simulink model "Arduino_observador_2021"  (R2021a)
settings: Solver=ode4  StartTime=0.0  StopTime=inf  FixedStep=0.001  RelTol=1e-3  EnableMultiTasking=on
values from neighbouring files (symbols this model uses):
  A = [-Ra/La -Kg/(Kt*La) ... (first row only)    [observador_arduino.m]
  B = [1/La ; 0]    [observador_arduino.m]
  C = [0 1]    [observador_arduino.m]
  K = [K1 K2]    [observador_arduino.m]
  ki = double(solve(coeffs_det_A_r(end-3)==pol_caract(4), ki))    [observador_arduino.m]
  L = place(A', C', desired_poles)'    [observador_arduino.m]
libraries: arduinolib x2
settings Model: SILPILModeSetting=veronly  ExtModeTrigDuration=2  Creator=lcauf  LastModifiedBy=carol
settings OptimizationCC: EnhancedBackFolding=on  PassReuseOutputArgsAs=Individual arguments  ZeroExternalMemoryAtStartup=off  ZeroInternalMemoryAtStartup=off  MaxStackSize=64  OptimizeBlockOrder=speed  DifferentSizesBufferReuse=on  OptimizationCustomize=off  EfficientTunableParamExpr=on
settings DebuggingCC: ParameterTunabilityLossMsg=error
settings HardwareCC: ProdBitPerPointer=32  ProdBitPerSizeT=32  ProdBitPerPtrDiffT=32  ProdLargestAtomicInteger=Long  ProdLargestAtomicFloat=Double  ProdWordSize=32  ProdHWDeviceType=ARM Compatible->ARM Cortex  UseEmbeddedCoderFeatures=off
settings SFSimCC: MATLABDynamicMemAlloc=off
settings RTWCC: SystemTargetFile=ert.tlc  HardwareBoard=Arduino Due  TemplateMakefile=ert_default_tmf  Toolchain=Arduino ARM  BuildConfiguration=Faster Runs
settings CodeAppCC: ForceParamTrailComments=on  IgnoreCustomStorageClasses=off  OperatorAnnotations=on  SimulinkDataObjDesc=on  SFDataObjDesc=on  InsertBlockDesc=on
settings ERTTargetCC: SupportContinuousTime=on  SupportNonInlinedSFcns=on  SupportVariableSizeSignals=on  ExtModeTransport=3  ExtModeStaticAlloc=on  ExtModeStaticAllocSize=24576  ExtModeMexFile=ext_xcp  ExtModeIntrfLevel=Level2 - Open

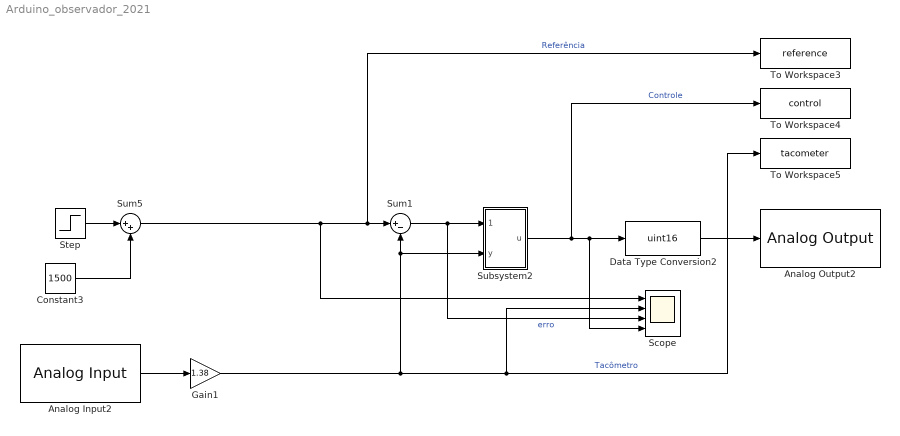
== system Arduino_observador_2021 ==
  Analog Input2 : arduinolib/Analog Input  pinNumber=1  ReadResultsOnly=off  ConversionTriggerSource=Software  ExternalTriggerType=uint32( 0 )  OutputDataType=uint16  EnableConversionCompleteNotify=off  EnableOuputStatus=off  SampleTime=-1  blockPlatform=arduino
  Analog Output2 : arduinolib/Analog Output  DACpin=DAC0  blockPlatform=arduino
      settings: SourceProductBaseCode=ARDUINO
  Constant3 : Constant  Value=1500
  Data Type Conversion2 : DataTypeConversion  OutDataTypeStr=uint16
  Gain1 : Gain  Gain=1.38
  Scope : Scope  NumInputPorts=4
  Step : Step  After=2000  SampleTime=0
  Subsystem2 : Subsystem
  Sum1 : Sum  Inputs=|+-
  Sum5 : Sum  Inputs=|++
  To Workspace3 : ToWorkspace  VariableName=reference  SaveFormat=Structure With Time  SampleTime=-1
  To Workspace4 : ToWorkspace  VariableName=control  SaveFormat=Structure With Time  SampleTime=-1
  To Workspace5 : ToWorkspace  VariableName=tacometer  SaveFormat=Structure With Time  SampleTime=-1
  wires:
  Sum1/1 -> Scope/3, Subsystem2/1(erro)  "erro"
  Analog Input2/1 -> Gain1/1
  Data Type Conversion2/1 -> Analog Output2/1
  Sum5/1 -> Scope/1, To Workspace3/1, Sum1/1  "Referência"
  Subsystem2/1(u) -> To Workspace4/1, Scope/4, Data Type Conversion2/1  "Controle"
  Constant3/1 -> Sum5/2
  Gain1/1 -> Scope/2, To Workspace5/1, Sum1/2, Subsystem2/2(y)  "Tacômetro"
  Step/1 -> Sum5/1

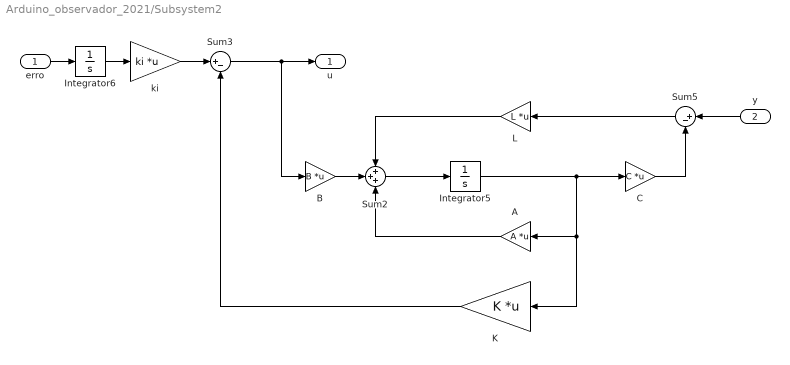
== system Arduino_observador_2021/Subsystem2 ==
  erro : Inport
  y : Inport  Port=2
  A : Gain  Gain=A  Multiplication=Matrix(K*u)
  B : Gain  Gain=B  Multiplication=Matrix(K*u)
  C : Gain  Gain=C  Multiplication=Matrix(K*u)
  Integrator5 : Integrator  InitialCondition=-2
  Integrator6 : Integrator
  K : Gain  Gain=K  Multiplication=Matrix(K*u)
  L : Gain  Gain=L  Multiplication=Matrix(K*u)
  Sum2 : Sum  Inputs=+++
  Sum3 : Sum  Inputs=|+-
  Sum5 : Sum  Inputs=|+-
  ki : Gain  Gain=ki  Multiplication=Matrix(K*u)
  u : Outport
  wires:
  K/1 -> Sum3/2
  Integrator6/1 -> ki/1
  y/1 -> Sum5/1
  erro/1 -> Integrator6/1
  Integrator5/1 -> C/1, K/1, A/1
  Sum5/1 -> L/1
  B/1 -> Sum2/2
  ki/1 -> Sum3/1
  Sum2/1 -> Integrator5/1
  C/1 -> Sum5/2
  Sum3/1 -> u/1, B/1
  A/1 -> Sum2/3
  L/1 -> Sum2/1
